simulink model "Subsystem2"  (R2020b)
settings: Solver=VariableStepAuto  StartTime=0.0  StopTime=10.0  RelTol=1e-3
settings Model: Creator=MY lenovo  LastModifiedBy=MY lenovo
settings DataIOCC: SaveOutput=off  SaveTime=off

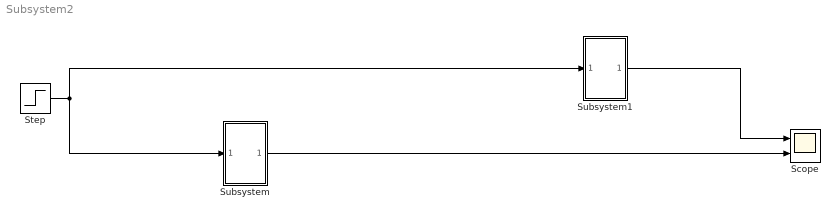
== system Subsystem2 ==
  Scope : Scope  NumInputPorts=2
  Step : Step  SampleTime=0
  Subsystem : Subsystem
  Subsystem1 : Subsystem
  wires:
  Step/1 -> Subsystem/1(In1), Subsystem1/1(In1)
  Subsystem1/1(Out1) -> Scope/1
  Subsystem/1(Out1) -> Scope/2

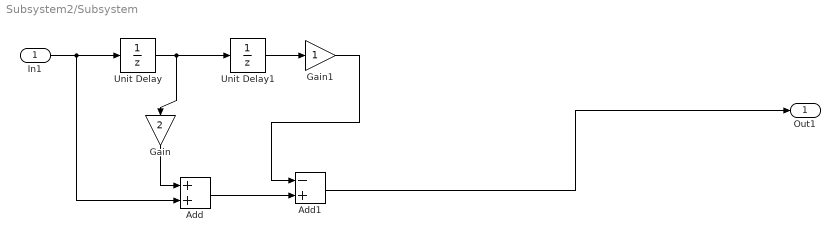
== system Subsystem2/Subsystem ==
  In1 : Inport
  Add : Sum
  Add1 : Sum  Inputs=-+
  Gain : Gain  Gain=2
  Gain1 : Gain
  Unit Delay : UnitDelay  SampleTime=-1  HasFrameUpgradeWarning=on
  Unit Delay1 : UnitDelay  SampleTime=-1  HasFrameUpgradeWarning=on
  Out1 : Outport
  wires:
  Add1/1 -> Out1/1
  In1/1 -> Unit Delay/1, Add/2
  Gain1/1 -> Add1/1
  Add/1 -> Add1/2
  Unit Delay/1 -> Gain/1, Unit Delay1/1
  Unit Delay1/1 -> Gain1/1
  Gain/1 -> Add/1

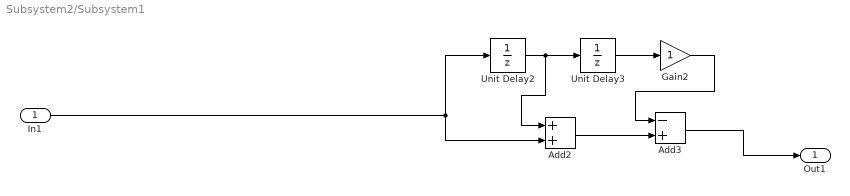
== system Subsystem2/Subsystem1 ==
  In1 : Inport
  Add2 : Sum
  Add3 : Sum  Inputs=-+
  Gain2 : Gain
  Unit Delay2 : UnitDelay  SampleTime=-1  HasFrameUpgradeWarning=on
  Unit Delay3 : UnitDelay  SampleTime=-1  HasFrameUpgradeWarning=on
  Out1 : Outport
  wires:
  Add3/1 -> Out1/1
  Unit Delay2/1 -> Unit Delay3/1, Add2/1
  Unit Delay3/1 -> Gain2/1
  Add2/1 -> Add3/2
  In1/1 -> Add2/2, Unit Delay2/1
  Gain2/1 -> Add3/1
